simulink model "Datos_exp"  (R2024b)
settings: Solver=VariableStepAuto  StartTime=0.0  StopTime=tmax  MaxStep=0.01  RelTol=1e-3
undefined symbols (not defined in the file): Beta, c, CI, idinput, Mu, Ts, V
libraries: simulink x1
settings Model: Creator=carlo  LastModifiedBy=USUARIO
settings DataIOCC: SaveOutput=off  SignalLogging=off  DSMLogging=off  SaveTime=off  ReturnWorkspaceOutputs=off
settings OptimizationCC: ReuseModelBlockBuffer=off
settings DebuggingCC: UnconnectedInputMsg=warning  UnconnectedOutputMsg=warning  UnconnectedLineMsg=warning
settings ModelReferenceCC: EnableRefExpFcnMdlSchedulingChecks=on
settings RTWCC: GPUComputeCapability=3.5  DLArmComputeVersion=19.05

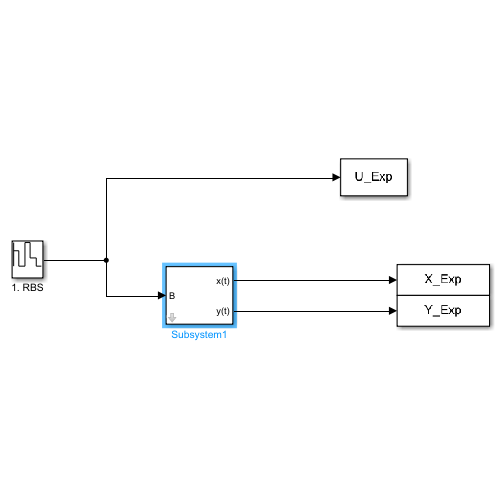
[thumbnail: Simulink's stored preview of the top-level diagram]
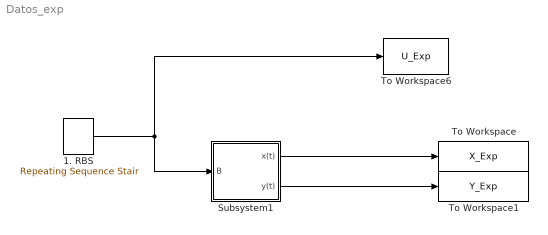
== system Datos_exp ==
  1. RBS : simulink/Sources/Repeating Sequence Stair  OutValues=idinput([2047, 1, 1], 'RBS', [0.01, 0.1], [600,800])  tsamp=Ts*5  OutMin=[]  OutMax=[]  OutDataTypeStr=double  OutputDataTypeScalingMode=double  OutDataType=fixdt(0,8)  ConRadixGroup=Best Precision: Vector-wise  OutScaling=2^-12
  Subsystem1 : Subsystem  mask{Beta=Beta, Mu=Mu, V=V, c=c, X0=CI}
      mask prompts: Beta "Tasa de Transmisión (Beta)"; Mu "Tasa de Muertes (Mu)"; V "Tasa de Recuperación (V)"; c "Contactos Suceptibles-Infectados (c)"; X0 "Suceptibles Iniciales (X0)"
  To Workspace : ToWorkspace  VariableName=X_Exp  SaveFormat=Structure With Time  SampleTime=Ts
  To Workspace1 : ToWorkspace  VariableName=Y_Exp  SaveFormat=Structure With Time  SampleTime=Ts
  To Workspace6 : ToWorkspace  VariableName=U_Exp  SaveFormat=Structure With Time  SampleTime=Ts
  wires:
  Subsystem1/1(x(t)) -> To Workspace/1
  Subsystem1/2(y(t)) -> To Workspace1/1
  1. RBS/1 -> Subsystem1/1(B), To Workspace6/1

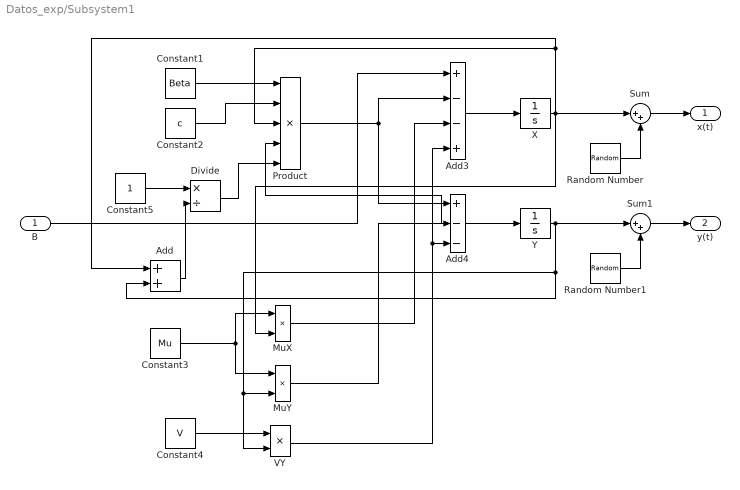
== system Datos_exp/Subsystem1 ==
  B : Inport
  Add : Sum
  Add3 : Sum  Inputs=+--+
  Add4 : Sum  Inputs=+--
  Constant1 : Constant  Value=Beta
  Constant2 : Constant  Value=c
  Constant3 : Constant  Value=Mu
  Constant4 : Constant  Value=V
  Constant5 : Constant
  Divide : Product  Inputs=*/
  MuX : Product
  MuY : Product
  Product : Product  Inputs=5
  Random Number : RandomNumber  Variance=64  SampleTime=Ts
  Random Number1 : RandomNumber  Variance=640  SampleTime=Ts
  Sum : Sum  Inputs=|++
  Sum1 : Sum  Inputs=|++
  VY : Product
  X : Integrator  InitialCondition=X0(1)  LimitOutput=on  LowerSaturationLimit=0
  Y : Integrator  InitialCondition=X0(2)  LimitOutput=on  LowerSaturationLimit=0
  x(t) : Outport
  y(t) : Outport  Port=2
  wires:
  X/1 -> Sum/1, Add/1, Product/3, MuX/2
  MuY/1 -> Add4/2
  Divide/1 -> Product/5
  Y/1 -> Sum1/1, Add/2, MuY/2, VY/2, Product/4
  Constant1/1 -> Product/1
  MuX/1 -> Add3/3
  Constant4/1 -> VY/1
  Add3/1 -> X/1
  Product/1 -> Add4/1, Add3/2
  Constant3/1 -> MuX/1, MuY/1
  B/1 -> Add3/1
  Add4/1 -> Y/1
  Constant2/1 -> Product/2
  Constant5/1 -> Divide/1
  VY/1 -> Add4/3, Add3/4
  Add/1 -> Divide/2
  Random Number/1 -> Sum/2
  Sum/1 -> x(t)/1
  Random Number1/1 -> Sum1/2
  Sum1/1 -> y(t)/1
